simulink model "controller"  (R2022b)
settings: Solver=FixedStepAuto  StartTime=0.0  StopTime=10.0  FixedStep=1/100  RelTol=1e-3
undefined symbols (not defined in the file): MAX_TORQUE, MAX_TORQUE_REVERSE
libraries: slpidlib x1
settings Model: Creator=DAUIN-Win10  LastModifiedBy=simon
settings DebuggingCC: UnconnectedInputMsg=warning  UnconnectedOutputMsg=warning  UnconnectedLineMsg=warning
settings ModelReferenceCC: EnableRefExpFcnMdlSchedulingChecks=on
settings RTWCC: DLArmComputeVersion=19.05

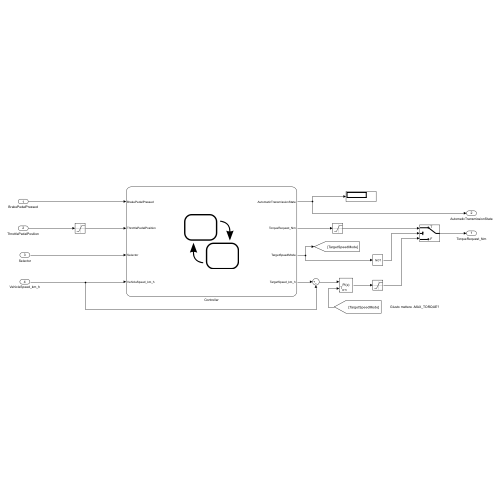
[thumbnail: Simulink's stored preview of the top-level diagram]
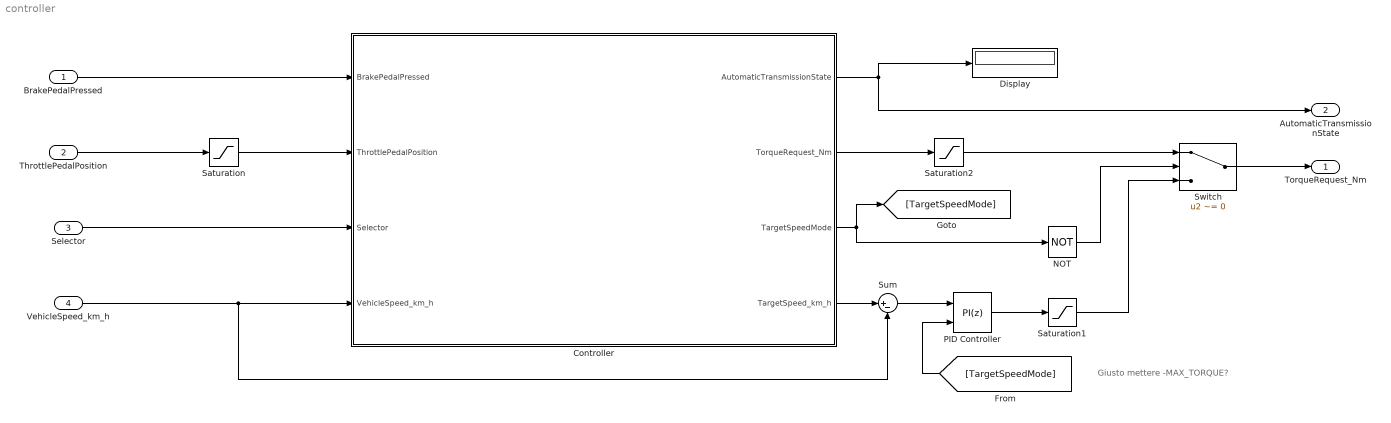
== system controller ==
  note: Giusto mettere -MAX_TORQUE?
  BrakePedalPressed : Inport  OutDataTypeStr=boolean
  ThrottlePedalPosition : Inport  Port=2  OutDataTypeStr=single
  Selector : Inport  Port=3  OutDataTypeStr=Enum: TransmissionState
  VehicleSpeed_km_h : Inport  Port=4  OutDataTypeStr=single  Unit=km/h
  Controller : Stateflow chart  TreatAsAtomicUnit=on
      settings: PortSchema="{\"entries\":[{\"content\":{\"sides\":[{\"content\":{\"connectorIds\":[\"In1\",\"In2\",\"In4\",\"In3\"]},\"type\":\"ConnectorPlacement.EquallySpacedRectSide\",\"uuid\":\"2f18118e-0843-4cb5-a956-6fbe9f973a93\"},{\"content\":{\"connectorIds\":[\"Out1\",\"Out2\",\"Out4\",\"Out3\"],\"side\":\"RIGHT\"},\"type\":\"ConnectorPlacement.EquallySpacedRectSide\",\"uuid\":\"8092894e-1a93-498e-82dc-1729ed135b0b\"},{\"content\":{\"connectorIds\":[],\"side\":\"TOP\"},\"type\":\"ConnectorPlacement.EquallySpacedRectSide\",\"uuid\":\"166517c2-1190-4c6d-a8f3-40e22d1b976e\"}]},\"type\":\"ConnectorPlacement.EquallySpacedConnector\",\"uuid\":\"ca5c1f38-53f7-468c-a97f-82447ab7a015\"}],\"packageUris\":[\"http://schema.mathworks.com/mf0/Connector/R2020b\"],\"version\":\"1.0\"}"
  Display : Display
  NOT : Logic  Operator=NOT  AllPortsSameDT=off  OutDataTypeStr=boolean
  PID Controller : slpidlib/PID Controller  Controller=PI  Form=Parallel  TimeDomain=Discrete-time  UseExternalTs=on  SampleTime=-1  IntegratorMethod=Forward Euler  FilterMethod=Forward Euler  ControllerParametersSource=internal  P=100  I=0.1  UseKiTs=off  D=1  N=100  UseFilter=on  TunerSelectOption=Transfer Function Based (PID Tuner App)  InitialConditionSource=internal  InitialConditionForIntegrator=0  InitialConditionForFilter=0  DifferentiatorICPrevScaledInput=0  ExternalReset=none  TrackingMode=off  Kt=1  LimitOutput=off  SatLimitsSource=internal  UpperSaturationLimit=inf  LowerSaturationLimit=-inf  LinearizeAsGain=on  AntiWindupMode=none  Kb=1  LimitIntegrator=off  UpperIntegratorSaturationLimit=inf  LowerIntegratorSaturationLimit=-inf  POutMin=[]  POutMax=[]  IOutMin=[]  IOutMax=[]  DOutMin=[]  DOutMax=[]  NOutMin=[]  NOutMax=[]  SumOutMin=[]  SumOutMax=[]  SaturationOutMin=[]  SaturationOutMax=[]  PParamMin=[]  PParamMax=[]  IParamMin=[]  IParamMax=[]  DParamMin=[]  DParamMax=[]  NParamMin=[]  NParamMax=[]  KbParamMin=[]  KbParamMax=[]  KtParamMin=[]  KtParamMax=[]  KbOutMin=[]  KbOutMax=[]  KtOutMin=[]  KtOutMax=[]  IntegratorOutMin=[]  IntegratorOutMax=[]  FilterOutMin=[]  FilterOutMax=[]  SumI1OutMin=[]  SumI1OutMax=[]  SumI2OutMin=[]  SumI2OutMax=[]  SumI3OutMin=[]  SumI3OutMax=[]  SumI4OutMin=[]  SumI4OutMax=[]  SumDOutMin=[]  SumDOutMax=[]  DifferentiatorOutMin=[]  DifferentiatorOutMax=[]  FilterDiffOutCoefMin=[]  FilterDiffOutCoefMax=[]  ReciprocalOutMin=[]  ReciprocalOutMax=[]  SumDenOutMin=[]  SumDenOutMax=[]  SumNumOutMin=[]  SumNumOutMax=[]  DivideOutMin=[]  DivideOutMax=[]  UdiffTsProdOutMin=[]  UdiffTsProdOutMax=[]  NTsProdOutMin=[]  NTsProdOutMax=[]  UintegralTsProdOutMin=[]  UintegralTsProdOutMax=[]  UngainTsProdOutMin=[]  UngainTsProdOutMax=[]  ClampingZeroOutDataTypeStr=Inherit: Inherit via back propagation  ClampingZeroOutMin=[]  ClampingZeroOutMax=[]  FilterDenConstantOutDataTypeStr=Inherit: Inherit via back propagation  FilterDenConstantOutMin=[]  FilterDenConstantOutMax=[]  PCopyOutDataTypeStr=Inherit: Inherit via back propagation  PCopyOutMin=[]  PCopyOutMax=[]  NCopyOutDataTypeStr=Inherit: Inherit via back propagation  NCopyOutMin=[]  NCopyOutMax=[]  IntegratorContinuousStateAttributes=''  IntegratorStateMustResolveToSignalObject=off  IntegratorRTWStateStorageClass=Auto  FilterContinuousStateAttributes=''  FilterStateMustResolveToSignalObject=off  FilterRTWStateStorageClass=Auto  ParallelPVariant=InternalParameters  IdealPVariant=Disabled  IVariant=InternalParameters  DVariant=Disabled  IntegratorVariant=Discrete  SatVariant=Disabled  AWVariant=Passthrough  PCopyVariant=Disabled  TRVariant=Disabled  FdbkBlocksVariant=Forward  IdealPFdbkVariant=Disabled  SatFdbkVariant=Disabled  DerivativeFilterVariant=Disabled  NVariant=Disabled  NCopyVariant=Disabled_SignalSpec  FilterICVariant=Disabled  IntegratorICVariant=InternalICs  ExternalResetVariant=Disabled  TRSumVariant=Passthrough  SumFdbkVariant=Disabled  SumVariant=Sum_PI  TsampFilterVariant=InternalTs  TsampNgainVariant=Passthrough  TsampIntegralVariant=ExternalTs  ExternalSaturationOutDataTypeStr=Inherit: Same as second input
  Saturation : Saturate  UpperLimit=1  LowerLimit=0  OutDataTypeStr=double
  Saturation1 : Saturate  UpperLimit=MAX_TORQUE  LowerLimit=-MAX_TORQUE
  Saturation2 : Saturate  UpperLimit=80  LowerLimit=-80
  Sum : Sum  Inputs=|+-
  Switch : Switch  Criteria=u2 ~= 0  SaturateOnIntegerOverflow=off  InputSameDT=off
  TorqueRequest_Nm : Outport  OutDataTypeStr=single  Unit=N*m
  AutomaticTransmissionState : Outport  Port=2  OutDataTypeStr=Enum: TransmissionState
  wires:
  Switch/1 -> TorqueRequest_Nm/1
  VehicleSpeed_km_h/1 -> Sum/2, Controller/3(VehicleSpeed_km_h)
  ThrottlePedalPosition/1 -> Saturation/1
  Saturation/1 -> Controller/2(ThrottlePedalPosition)
  Selector/1 -> Controller/4(Selector)
  BrakePedalPressed/1 -> Controller/1(BrakePedalPressed)
  Controller/2(TorqueRequest_Nm) -> Saturation2/1
  Controller/1(AutomaticTransmissionState) -> AutomaticTransmissionState/1, Display/1
  Controller/4(TargetSpeedMode) -> NOT/1, [TargetSpeedMode]
  Saturation2/1 -> Switch/1
  NOT/1 -> Switch/2
  Controller/3(TargetSpeed_km_h) -> Sum/1
  PID Controller/1 -> Saturation1/1
  Saturation1/1 -> Switch/3
  Sum/1 -> PID Controller/1
  [TargetSpeedMode] -> PID Controller/2

== stateflow chart controller/Controller ==
  state Brake_mode
    entry:
    AutomaticTransmissionState = TransmissionState(4);
    state CarStopped
      entry:
      TargetSpeed_km_h = 0;
      TargetSpeedMode = 1;
      exit:
      TargetSpeedMode = 0;
      TorqueRequest_Nm = 0;
    state Acceleration
      during:
      TorqueRequest_Nm = MAX_TORQUE*...
      3/2*(ThrottlePedalPosition-1/3);
    state RegenerativeBreaking
      during:
      TorqueRequest_Nm = -MAX_TORQUE*...
      (1-3*ThrottlePedalPosition);
    (default) -> (junction 178)
    (junction 178) -> CarStopped [order 2] : [abs(VehicleSpeed_km_h) <= 0.5 &&...
        |  ThrottlePedalPosition <= 1/3 ]
    (junction 178) -> Acceleration [order 3]
    (junction 178) -> Acceleration [order 1] : [ThrottlePedalPosition > 1/3]
    CarStopped -> Acceleration : [ThrottlePedalPosition > 1/3]
    RegenerativeBreaking -> CarStopped [order 2] : [VehicleSpeed_km_h <= 0.5]
    Acceleration -> RegenerativeBreaking : [ThrottlePedalPosition <= 1/3 ]
    RegenerativeBreaking -> Acceleration [order 1] : [ThrottlePedalPosition > 1/3 ]
  note: Qua aggiungerei la spiegazione delle transizioni che escono da Brake_pedal_pressed potrebbe non capire
  state Brake_pedal_pressed
    state Released
      entry:
      TargetSpeedMode = 1;
      exit:
      TargetSpeedMode = 0;
    state Pressed
      entry:
      TorqueRequest_Nm = 0;
    (default) -> Pressed
    Pressed -> Released : [BrakePedalPressed == false && ...
        | abs(VehicleSpeed_km_h) <= 0.5]
    Released -> Pressed : [BrakePedalPressed == true]
  note: Park(0)
      | Reverse(1)
      | Neutral(2)
      | Drive(3)
      | Brake(4)
  state Drive_mode
    entry:
    AutomaticTransmissionState = TransmissionState(3);
    during:
    TorqueRequest_Nm = MAX_TORQUE*ThrottlePedalPosition;
  state Park_mode
    entry:
    AutomaticTransmissionState = TransmissionState(0);
    TargetSpeedMode = 0;
    TargetSpeed_km_h = 0;
    during:
    TorqueRequest_Nm = 0;
  state Neutral_mode
    entry:
    AutomaticTransmissionState = TransmissionState(2);
    during:
    TorqueRequest_Nm = 0;
  state Reverse_mode
    entry:
    AutomaticTransmissionState = TransmissionState(1);
    during:
    TorqueRequest_Nm = -1*MAX_TORQUE_REVERSE*ThrottlePedalPosition;
  Brake_pedal_pressed -> Brake_mode [order 3] : [(AutomaticTransmissionState == 4 ...
      | && ThrottlePedalPosition > 1/3 ...
      | && BrakePedalPressed == false )]
  Brake_mode -> Brake_pedal_pressed [order 2] : [BrakePedalPressed == true]
      | {TargetSpeed_km_h = 5}
  Brake_mode -> Drive_mode [order 1] : [Selector ~= 4]
  Drive_mode -> Brake_mode [order 2] : [Selector == 4 && (ThrottlePedalPosition > 1/3  || abs(VehicleSpeed_km_h) <= 0.5)]
  Brake_pedal_pressed -> Reverse_mode [order 4] : [(AutomaticTransmissionState == 1 &&...
      |  ThrottlePedalPosition > 0 ...
      |  && BrakePedalPressed == false )]
  Reverse_mode -> Brake_pedal_pressed [order 2] : [BrakePedalPressed == true]
      | {TargetSpeed_km_h = -5}
  Brake_pedal_pressed -> Neutral_mode [order 2] : [(Selector <= 2 && AutomaticTransmissionState == 3) ||...
      | (Selector > 1 && AutomaticTransmissionState == 1)]
  Brake_pedal_pressed -> Drive_mode [order 1] : [(Selector <= 3 && AutomaticTransmissionState == 4)...
      | || (AutomaticTransmissionState == 3 &&...
      |  ThrottlePedalPosition > 0 ...
      |  && BrakePedalPressed == false )]
  Drive_mode -> Brake_pedal_pressed [order 3] : [BrakePedalPressed == true]
      | {TargetSpeed_km_h = 5}
  (default) -> Park_mode
  Drive_mode -> Neutral_mode [order 1] : [Selector <= 2]
  Neutral_mode -> Drive_mode [order 1] : [Selector >= 3 && VehicleSpeed_km_h > -5 && BrakePedalPressed]
  Park_mode -> Neutral_mode : [Selector ~= 0 && BrakePedalPressed]
  Neutral_mode -> Park_mode [order 3] : [Selector == 0 && abs(VehicleSpeed_km_h) < 5 ...
      | && BrakePedalPressed]
  Reverse_mode -> Neutral_mode [order 1] : [Selector ~= 1]
  Neutral_mode -> Reverse_mode [order 2] : [Selector == 1 && VehicleSpeed_km_h < 5 && BrakePedalPressed]
  data: BrakePedalPressed input; ThrottlePedalPosition input; VehicleSpeed_km_h input; AutomaticTransmissionState output; TorqueRequest_Nm output; MAX_TORQUE parameter; MAX_TORQUE_REVERSE parameter; TargetSpeed_km_h output; TargetSpeedMode output; Selector input
